simulink model "Final_EV_Model"  (R2020b)
settings: Solver=VariableStepAuto  StartTime=0.0  StopTime=2000  RelTol=1e-3
model workspace (MAT data in the model file):
  SoC_initial = Simulink.Parameter
  SoC_initial.DataType = 'auto'
  SoC_initial.Dimensions = [0 0]
values from neighbouring files (symbols this model uses):
  eff1 = [65 65 65 65 65 65 65 65 65 65 65 65 ... (600000 elements, 12000x50)]    [Frid27May_Data.mat]
  eff2 = [78 78 78 78 78 78 78 78 78 78 78 78 ... (600000 elements, 12000x50)]    [Frid27May_Data.mat]
  eff3 = [78 78 78 78 78 78 78 78 78 78 78 78 ... (600000 elements, 12000x50)]    [Frid27May_Data.mat]
  eff4 = [78 78 78 78 78 78 78 78 78 78 78 78 ... (600000 elements, 12000x50)]    [Frid27May_Data.mat]
  eff5 = [76 76 76 76 76 76 76 76 76 76 76 76 ... (600000 elements, 12000x50)]    [Frid27May_Data.mat]
  speed = [1 2 3 4 5 6 7 8 9 10 11 12 ... (12000 elements, 1x12000)]    [Frid27May_Data.mat]
  torque1 = [1 2 3 4 5 6 7 8 9 10 11 12 ... (50 elements, 1x50)]    [Frid27May_Data.mat]
  torque2 = [51 52 53 54 55 56 57 58 59 60 61 62 ... (50 elements, 1x50)]    [Frid27May_Data.mat]
  torque3 = [101 102 103 104 105 106 107 108 109 110 111 112 ... (50 elements, 1x50)]    [Frid27May_Data.mat]
  torque4 = [151 152 153 154 155 156 157 158 159 160 161 162 ... (50 elements, 1x50)]    [Frid27May_Data.mat]
  torque5 = [201 202 203 204 205 206 207 208 209 210 211 212 ... (50 elements, 1x50)]    [Frid27May_Data.mat]
undefined symbols (not defined in the file or in its folder): temp_inside, temp_outside
libraries: drivingcycle_lib x2, pid_lib x1
settings Model: Creator=joshuaafengbai  LastModifiedBy=joshuaafengbai

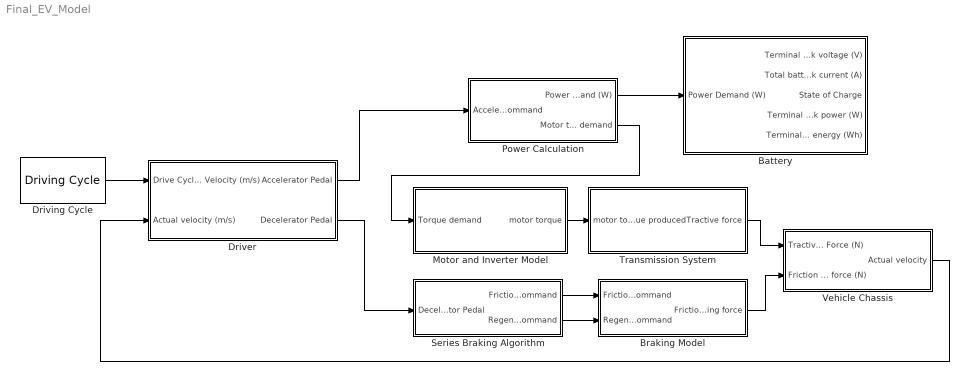
== system Final_EV_Model ==
  Battery : Subsystem
  Braking Model : Subsystem
  "Driver " : Subsystem
  Driving Cycle : drivingcycle_lib/Driving Cycle  CycleName=NEDC  CycleRepeatsForever=off
      settings: SourceProductName=Driving Cycle Blockset
  Motor and Inverter Model : Subsystem
  Power Calculation : Subsystem
  Series Braking Algorithm : Subsystem
  Transmission System : Subsystem
  Vehicle Chassis : Subsystem
  wires:
  Motor and Inverter Model/1(motor torque) -> Transmission System/1(motor torque produced)
  Transmission System/1(Tractive force) -> Vehicle Chassis/1(Tractive Force (N))
  "Driver "/1(Accelerator Pedal) -> Power Calculation/1(Acceleration command)
  Vehicle Chassis/1(Actual velocity) -> "Driver "/2(Actual velocity (m/s))
  Driving Cycle/2 -> "Driver "/1(Drive Cycle Velocity (m/s))
  "Driver "/2(Decelerator Pedal) -> Series Braking Algorithm/1(Decelerator Pedal)
  Series Braking Algorithm/1(" Friction brake command") -> Braking Model/1(Friction command)
  Series Braking Algorithm/2(Regen brake command) -> Braking Model/2(Regen command)
  Power Calculation/1(Power Demand (W)) -> Battery/1(Power Demand (W))
  Power Calculation/2(Motor torque demand) -> Motor and Inverter Model/1(Torque demand)
  Braking Model/1(Friction braking force) -> Vehicle Chassis/2(Friction braking force (N))

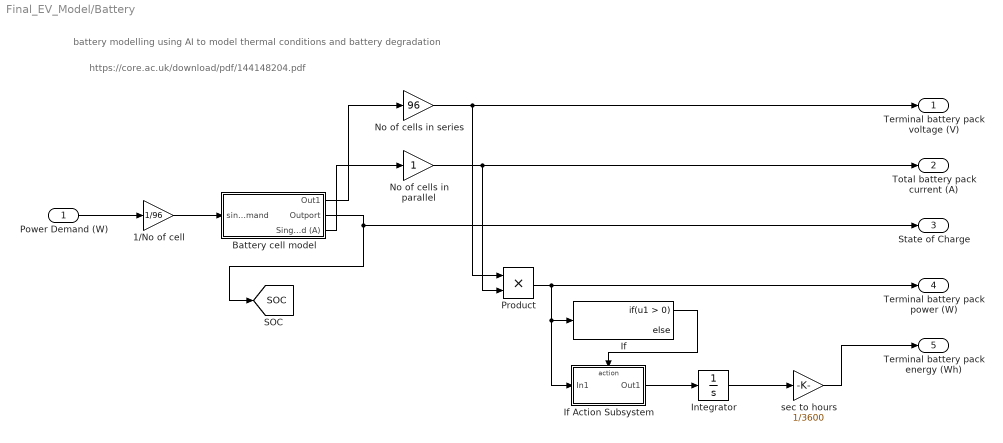
== system Final_EV_Model/Battery ==
  note: battery modelling using AI to model thermal conditions and battery degradation
  note: https://core.ac.uk/download/pdf/144148204.pdf
  Power Demand (W) : Inport
  1/No of cell : Gain  Gain=1/96
  Battery cell model : Subsystem
  If : If
  If Action Subsystem : Subsystem  TreatAsAtomicUnit=on
  Integrator : Integrator
  No of cells in parallel : Gain
  No of cells in series : Gain  Gain=96
  Product : Product
  sec to hours : Gain  Gain=1/3600
  Terminal battery pack voltage (V) : Outport
  Total battery pack current (A) : Outport  Port=2
  State of Charge : Outport  Port=3
  Terminal battery pack power (W) : Outport  Port=4
  Terminal battery pack energy (Wh) : Outport  Port=5
  tag scope: SOC=global
  wires:
  No of cells in series/1 -> Product/1, Terminal battery pack voltage (V)/1
  No of cells in parallel/1 -> Total battery pack current (A)/1, Product/2
  Product/1 -> If/1, If Action Subsystem/1(In1), Terminal battery pack power (W)/1
  sec to hours/1 -> Terminal battery pack energy (Wh)/1
  Integrator/1 -> sec to hours/1
  1/No of cell/1 -> Battery cell model/1(single cell power demand)
  Battery cell model/1(Out1) -> No of cells in series/1
  Battery cell model/2(Outport) -> State of Charge/1, [SOC]
  Power Demand (W)/1 -> 1/No of cell/1
  Battery cell model/3(Single cell current demand (A)) -> No of cells in parallel/1
  If/1 -> If Action Subsystem/Action
  If Action Subsystem/1(Out1) -> Integrator/1

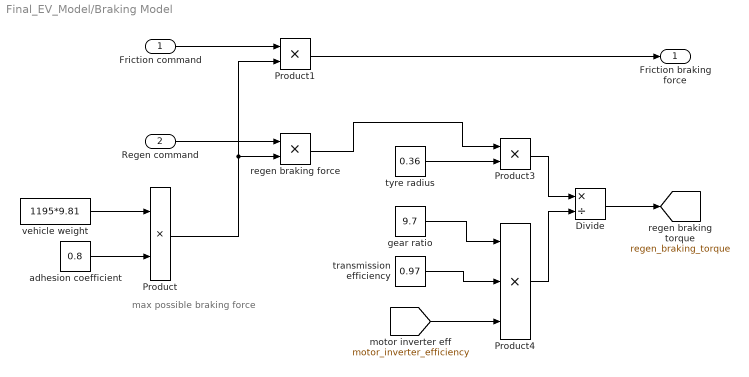
== system Final_EV_Model/Braking Model ==
  note: max possible
      | braking force
  Friction command : Inport
  Regen command : Inport  Port=2
  Divide : Product  Inputs=*/
  Product : Product
  Product1 : Product
  Product3 : Product
  Product4 : Product  Inputs=3
  adhesion coefficient : Constant  Value=0.8
  gear ratio : Constant  Value=9.7
  regen braking force : Product
  transmission efficiency : Constant  Value=0.97
  tyre radius : Constant  Value=0.36
  vehicle weight : Constant  Value=1195*9.81
  Friction braking force : Outport
  tag scope: regen_braking_torque=global
  wires:
  vehicle weight/1 -> Product/1
  adhesion coefficient/1 -> Product/2
  Product1/1 -> Friction braking force/1
  regen braking force/1 -> Product3/1
  Product/1 -> Product1/2, regen braking force/2
  Friction command/1 -> Product1/1
  Regen command/1 -> regen braking force/1
  tyre radius/1 -> Product3/2
  gear ratio/1 -> Product4/1
  transmission efficiency/1 -> Product4/2
  Product3/1 -> Divide/1
  Product4/1 -> Divide/2
  Divide/1 -> [regen_braking_torque]
  [motor_inverter_efficiency] -> Product4/3

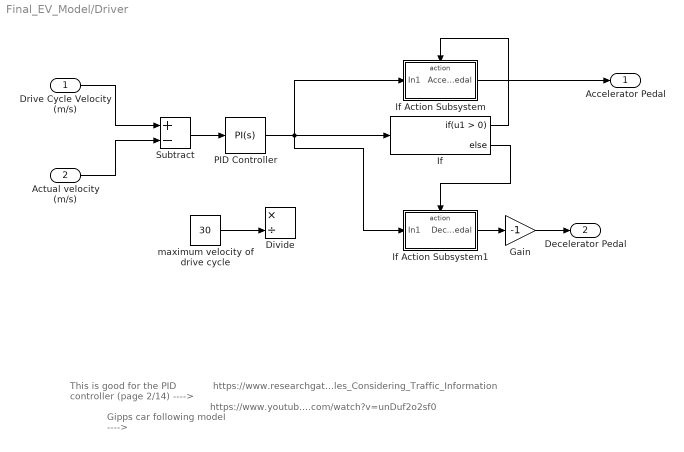
== system Final_EV_Model/Driver  ==
  note: Gipps car following model ---->
  note: https://www.youtube.com/watch?v=unDuf2o2sf0
  note: This is good for the PID controller (page 2/14) ---->
  note: https://www.researchgate.net/publication/335954963_Research_on_the_Energy-Saving_Strategy_of_Path_Planning_for_Electric_Vehicles_Considering_Traffic_Information
  Drive Cycle Velocity (m/s) : Inport
  Actual velocity (m/s) : Inport  Port=2
  Divide : Product  Inputs=*/
  Gain : Gain  Gain=-1
  If : If
  If Action Subsystem : Subsystem  TreatAsAtomicUnit=on
  If Action Subsystem1 : Subsystem  TreatAsAtomicUnit=on
  PID Controller : pid_lib/PID Controller  Controller=PI  Form=Parallel  TimeDomain=Continuous-time  UseExternalTs=off  SampleTime=-1  IntegratorMethod=Forward Euler  FilterMethod=Forward Euler  ControllerParametersSource=internal  P=10  I=1  D=0  UseFilter=on  N=1  TunerSelectOption=Transfer Function Based (PID Tuner App)  InitialConditionSource=internal  InitialConditionForIntegrator=0  InitialConditionForFilter=0  DifferentiatorICPrevScaledInput=0  ExternalReset=none  TrackingMode=off  Kt=1  LimitOutput=off  SatLimitsSource=internal  UpperSaturationLimit=inf  LowerSaturationLimit=-inf  LinearizeAsGain=on  AntiWindupMode=none  Kb=1  POutMin=[]  POutMax=[]  IOutMin=[]  IOutMax=[]  DOutMin=[]  DOutMax=[]  NOutMin=[]  NOutMax=[]  SumOutMin=[]  SumOutMax=[]  SaturationOutMin=[]  SaturationOutMax=[]  PParamMin=[]  PParamMax=[]  IParamMin=[]  IParamMax=[]  DParamMin=[]  DParamMax=[]  NParamMin=[]  NParamMax=[]  KbParamMin=[]  KbParamMax=[]  KtParamMin=[]  KtParamMax=[]  KbOutMin=[]  KbOutMax=[]  KtOutMin=[]  KtOutMax=[]  IntegratorOutMin=[]  IntegratorOutMax=[]  FilterOutMin=[]  FilterOutMax=[]  SumI1OutMin=[]  SumI1OutMax=[]  SumI2OutMin=[]  SumI2OutMax=[]  SumI3OutMin=[]  SumI3OutMax=[]  SumI4OutMin=[]  SumI4OutMax=[]  SumDOutMin=[]  SumDOutMax=[]  DifferentiatorOutMin=[]  DifferentiatorOutMax=[]  FilterDiffOutCoefMin=[]  FilterDiffOutCoefMax=[]  ReciprocalOutMin=[]  ReciprocalOutMax=[]  SumDenOutMin=[]  SumDenOutMax=[]  SumNumOutMin=[]  SumNumOutMax=[]  DivideOutMin=[]  DivideOutMax=[]  UdiffTsProdOutMin=[]  UdiffTsProdOutMax=[]  NTsProdOutMin=[]  NTsProdOutMax=[]  UintegralTsProdOutMin=[]  UintegralTsProdOutMax=[]  UngainTsProdOutMin=[]  UngainTsProdOutMax=[]  IntegratorContinuousStateAttributes=''  IntegratorStateMustResolveToSignalObject=off  IntegratorRTWStateStorageClass=Auto  FilterContinuousStateAttributes=''  FilterStateMustResolveToSignalObject=off  FilterRTWStateStorageClass=Auto  ParallelPVariant=InternalParameters  IdealPVariant=Disabled  IVariant=InternalParameters  DVariant=Disabled  IntegratorVariant=Continuous  SatVariant=Disabled  AWVariant=Passthrough  PCopyVariant=Disabled  TRVariant=Disabled  FdbkBlocksVariant=Forward  IdealPFdbkVariant=Disabled  SatFdbkVariant=Disabled  DerivativeFilterVariant=Disabled  NVariant=Disabled  NCopyVariant=Disabled_SignalSpec  FilterICVariant=Disabled  IntegratorICVariant=InternalICs  ExternalResetVariant=Disabled  TRSumVariant=Passthrough  SumFdbkVariant=Disabled  SumVariant=Sum_PI  TsampFilterVariant=InternalTs  TsampNgainVariant=Passthrough  TsampIntegralVariant=Passthrough  ExternalSaturationOutDataTypeStr=Inherit: Same as second input
  Subtract : Sum  Inputs=+-
  maximum velocity of drive cycle : Constant  Value=30
  Accelerator Pedal : Outport
  Decelerator Pedal : Outport  Port=2
  wires:
  Drive Cycle Velocity (m/s)/1 -> Subtract/1
  Actual velocity (m/s)/1 -> Subtract/2
  Subtract/1 -> PID Controller/1
  If/1 -> If Action Subsystem/Action
  If/2 -> If Action Subsystem1/Action
  maximum velocity of drive cycle/1 -> Divide/2
  If Action Subsystem/1(Accelerator Pedal) -> Accelerator Pedal/1
  PID Controller/1 -> If/1, If Action Subsystem/1(In1), If Action Subsystem1/1(In1)
  If Action Subsystem1/1(Decelerator Pedal) -> Gain/1
  Gain/1 -> Decelerator Pedal/1

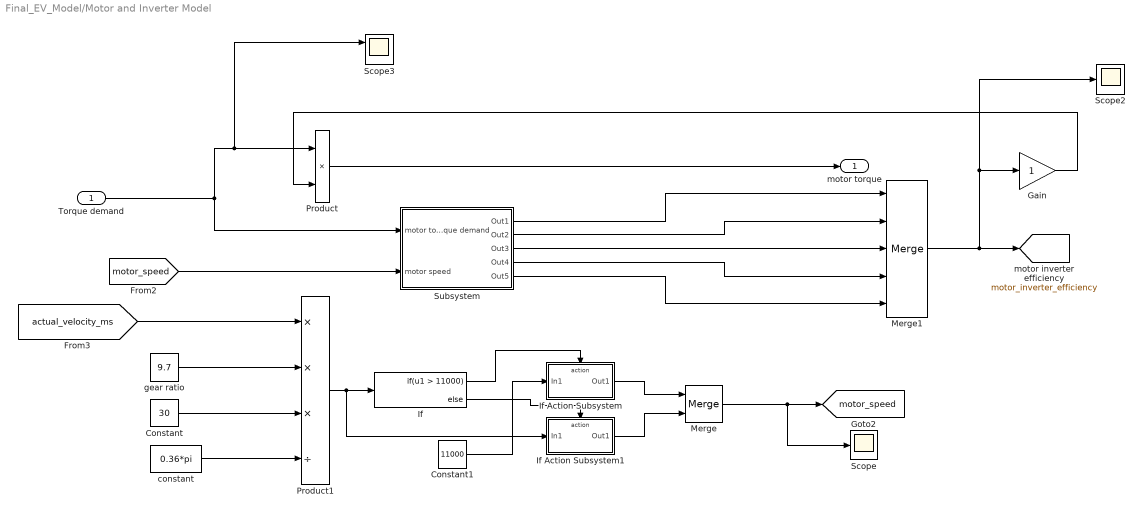
== system Final_EV_Model/Motor and Inverter Model ==
  Torque demand : Inport
  Constant : Constant  Value=30
  Constant1 : Constant  Value=11000
  Gain : Gain
  If : If  IfExpression=u1 > 11000
  If Action Subsystem : Subsystem  TreatAsAtomicUnit=on
  If Action Subsystem1 : Subsystem  TreatAsAtomicUnit=on
  Merge : Merge
  Merge1 : Merge  Inputs=5
  Product : Product
  Product1 : Product  Inputs=***/
  Scope : Scope
  Scope2 : Scope
  Scope3 : Scope  NumInputPorts=2
  Subsystem : Subsystem
  constant : Constant  Value=0.36*pi
  gear ratio : Constant  Value=9.7
  motor torque : Outport
  tag scope: motor_inverter_efficiency=global, motor_speed=global
  wires:
  Merge1/1 -> Scope2/1, Gain/1, [motor_inverter_efficiency]
  Product/1 -> motor torque/1
  [actual_velocity_ms] -> Product1/1
  gear ratio/1 -> Product1/2
  Torque demand/1 -> Scope3/1, Product/1, Subsystem/1(motor torque demand)
  [motor_speed] -> Subsystem/2(motor speed)
  Subsystem/1(Out1) -> Merge1/1
  Subsystem/2(Out2) -> Merge1/2
  Subsystem/3(Out3) -> Merge1/3
  Subsystem/4(Out4) -> Merge1/4
  Subsystem/5(Out5) -> Merge1/5
  Constant/1 -> Product1/3
  constant/1 -> Product1/4
  If/1 -> If Action Subsystem/Action
  Product1/1 -> If Action Subsystem1/1(In1), If/1
  Constant1/1 -> If Action Subsystem/1(In1)
  If/2 -> If Action Subsystem1/Action
  If Action Subsystem/1(Out1) -> Merge/1
  If Action Subsystem1/1(Out1) -> Merge/2
  Merge/1 -> Scope/1, [motor_speed]
  Gain/1 -> Product/2

== system Final_EV_Model/Power Calculation ==
  Acceleration command : Inport
  Add : Sum
  Add1 : Sum  Inputs=-+
  Gain : Gain  Gain=3/5
  Product : Product
  Scope : Scope
  auxillary system power demand : Subsystem
  driving power demand : Subsystem
  max available torque (Nm) : Constant  Value=250
  Power Demand (W) : Outport
  Motor torque demand : Outport  Port=2
  wires:
  Add/1 -> Power Demand (W)/1
  Acceleration command/1 -> Product/2
  Product/1 -> Motor torque demand/1, Add1/2
  auxillary system power demand/1(Power Demand (W)) -> Add/1
  Add1/1 -> driving power demand/1(Torque demand (Nm))
  driving power demand/1(power demand (W)) -> Add/2
  max available torque (Nm)/1 -> Product/1
  [regen_braking_torque] -> Gain/1
  Gain/1 -> Scope/1, Add1/1

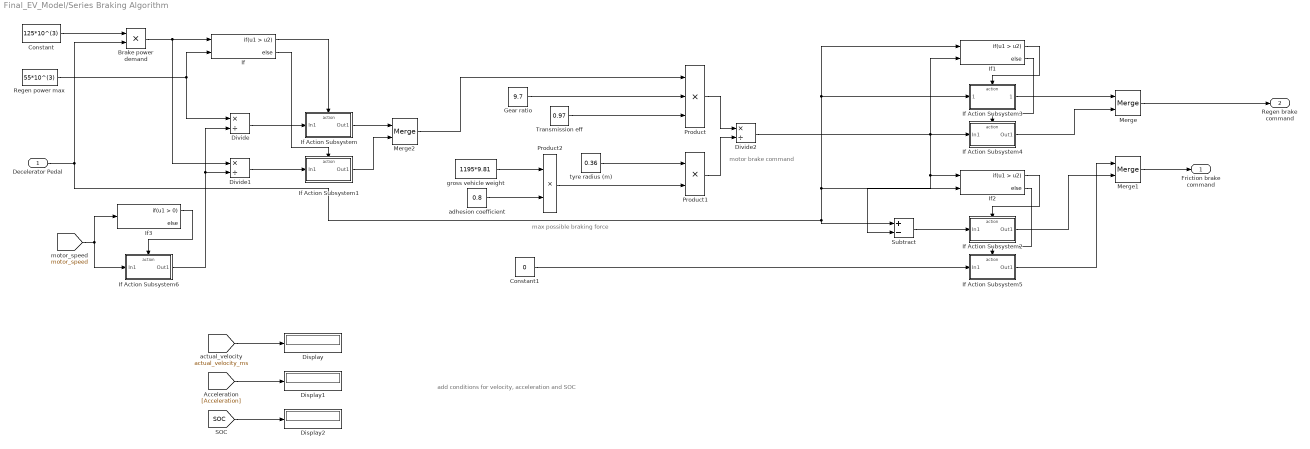
== system Final_EV_Model/Series Braking Algorithm ==
  note: add conditions for velocity, acceleration and SOC
  note: motor brake
      | command
  note: max possible
      | braking force
  Decelerator Pedal : Inport
  Brake power demand : Product
  Constant : Constant  Value=125*10^(3)
  Constant1 : Constant  Value=0
  Display : Display
  Display1 : Display
  Display2 : Display
  Divide : Product  Inputs=*/
  Divide1 : Product  Inputs=*/
  Divide2 : Product  Inputs=*/
  Gear ratio : Constant  Value=9.7
  If : If  NumInputs=2  IfExpression=u1 > u2
  If Action Subsystem : Subsystem  TreatAsAtomicUnit=on
  If Action Subsystem1 : Subsystem  TreatAsAtomicUnit=on
  If Action Subsystem2 : Subsystem  TreatAsAtomicUnit=on
  If Action Subsystem3 : Subsystem  TreatAsAtomicUnit=on
  If Action Subsystem4 : Subsystem  TreatAsAtomicUnit=on
  If Action Subsystem5 : Subsystem  TreatAsAtomicUnit=on
  If Action Subsystem6 : Subsystem  TreatAsAtomicUnit=on
  If1 : If  NumInputs=2  IfExpression=u1 > u2
  If2 : If  NumInputs=2  IfExpression=u1 > u2
  If3 : If
  Merge : Merge
  Merge1 : Merge
  Merge2 : Merge
  Product : Product  Inputs=3
  Product1 : Product
  Product2 : Product
  Regen power max : Constant  Value=55*10^(3)
  Subtract : Sum  Inputs=+-
  Transmission eff : Constant  Value=0.97
  adhesion coefficient : Constant  Value=0.8
  gross vehicle weight : Constant  Value=1195*9.81
  tyre radius (m) : Constant  Value=0.36
  " Friction brake command" : Outport
  Regen brake command : Outport  Port=2
  wires:
  Regen power max/1 -> Divide/1, If/2
  Brake power demand/1 -> If/1, Divide1/1
  If/1 -> If Action Subsystem/Action
  [motor_speed] -> If Action Subsystem6/1(In1), If3/1
  Divide/1 -> If Action Subsystem/1(In1)
  If/2 -> If Action Subsystem1/Action
  Divide1/1 -> If Action Subsystem1/1(In1)
  Gear ratio/1 -> Product/2
  Transmission eff/1 -> Product/3
  tyre radius (m)/1 -> Product1/1
  gross vehicle weight/1 -> Product2/1
  Product2/1 -> Product1/2
  adhesion coefficient/1 -> Product2/2
  Product/1 -> Divide2/1
  Product1/1 -> Divide2/2
  Decelerator Pedal/1 -> If1/1, If Action Subsystem3/1(Decelerator Pedal), If2/2, Subtract/1, Brake power demand/2
  Divide2/1 -> If1/2, If2/1, Subtract/2, If Action Subsystem4/1(In1)
  If1/1 -> If Action Subsystem3/Action
  If Action Subsystem3/1(Regen brake command) -> Merge/1
  If1/2 -> If Action Subsystem4/Action
  Constant1/1 -> If Action Subsystem5/1(In1)
  Subtract/1 -> If Action Subsystem2/1(In1)
  If Action Subsystem4/1(Out1) -> Merge/2
  If Action Subsystem5/1(Out1) -> Merge1/1
  If Action Subsystem2/1(Out1) -> Merge1/2
  Merge1/1 -> " Friction brake command"/1
  If Action Subsystem/1(Out1) -> Merge2/1
  If Action Subsystem1/1(Out1) -> Merge2/2
  Merge2/1 -> Product/1
  If2/1 -> If Action Subsystem2/Action
  If2/2 -> If Action Subsystem5/Action
  Constant/1 -> Brake power demand/1
  [SOC] -> Display2/1
  [Acceleration] -> Display1/1
  [actual_velocity_ms] -> Display/1
  If3/1 -> If Action Subsystem6/Action
  If Action Subsystem6/1(Out1) -> Divide1/2, Divide/2
  Merge/1 -> Regen brake command/1

== system Final_EV_Model/Transmission System ==
  motor torque produced : Inport
  Divide : Product  Inputs=*/
  Product : Product  Inputs=3
  Single speed gear ratio : Constant  Value=9.7
  dynamic tyre radius : Constant  Value=0.36
  transmission efficiency : Constant  Value=0.97
  Tractive force : Outport
  wires:
  motor torque produced/1 -> Product/1
  Single speed gear ratio/1 -> Product/2
  transmission efficiency/1 -> Product/3
  Product/1 -> Divide/1
  dynamic tyre radius/1 -> Divide/2
  Divide/1 -> Tractive force/1

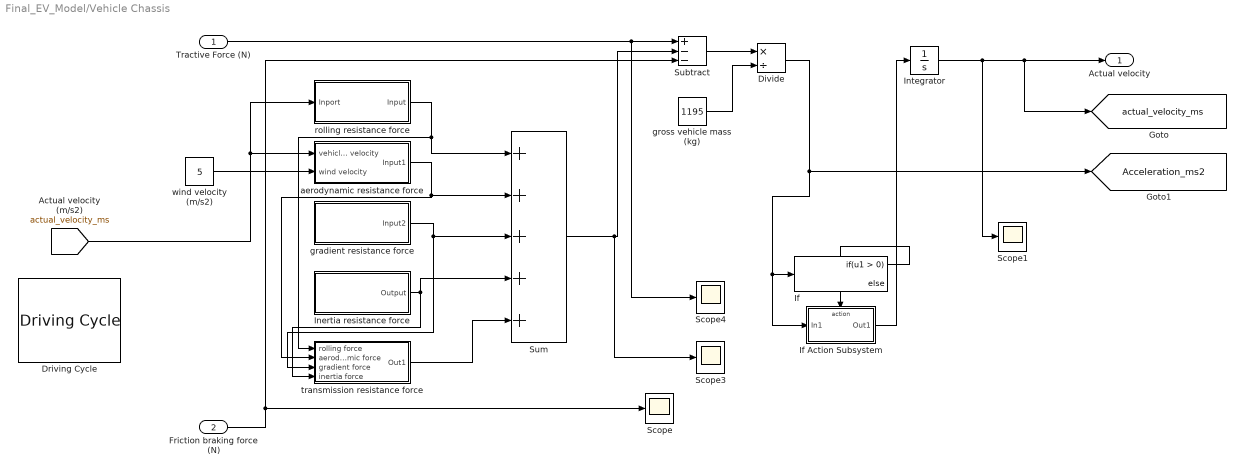
== system Final_EV_Model/Vehicle Chassis ==
  Tractive Force (N) : Inport
  Friction braking force (N) : Inport  Port=2
  Divide : Product  Inputs=*/
  Driving Cycle : drivingcycle_lib/Driving Cycle  CycleName=NEDC  CycleRepeatsForever=off
      settings: SourceProductName=Driving Cycle Blockset
  If : If
  If Action Subsystem : Subsystem  TreatAsAtomicUnit=on
  Inertia resistance force : Subsystem
  Integrator : Integrator
  Scope{,1,3..4} (4 alike) : Scope
  Subtract : Sum  Inputs=+--
  Sum : Sum  Inputs=5
  aerodynamic resistance force : Subsystem
  gradient resistance force : Subsystem
  gross vehicle mass (kg) : Constant  Value=1195
  rolling resistance force : Subsystem
  transmission resistance force : Subsystem
  wind velocity (m/s2) : Constant  Value=5
  Actual velocity : Outport
  tag scope: Acceleration_ms2=global, actual_velocity_ms=global
  wires:
  rolling resistance force/1(Input) -> Sum/1, transmission resistance force/1(rolling force)
  aerodynamic resistance force/1(Input1) -> transmission resistance force/2(aerodynamic force), Sum/2
  gradient resistance force/1(Input2) -> Sum/3, transmission resistance force/3(gradient force)
  Inertia resistance force/1(Output) -> Sum/4, transmission resistance force/4(inertia force)
  transmission resistance force/1(Out1) -> Sum/5
  Sum/1 -> Scope3/1, Subtract/2
  Subtract/1 -> Divide/1
  gross vehicle mass (kg)/1 -> Divide/2
  Divide/1 -> If Action Subsystem/1(In1), If/1, [Acceleration_ms2]
  Integrator/1 -> Scope1/1, [actual_velocity_ms], Actual velocity/1
  Friction braking force (N)/1 -> Scope/1, Subtract/3
  Tractive Force (N)/1 -> Scope4/1, Subtract/1
  wind velocity (m/s2)/1 -> aerodynamic resistance force/2(wind velocity)
  [actual_velocity_ms] -> rolling resistance force/1(Inport), aerodynamic resistance force/1(vehicle velocity)
  If/1 -> If Action Subsystem/Action
  If Action Subsystem/1(Out1) -> Integrator/1

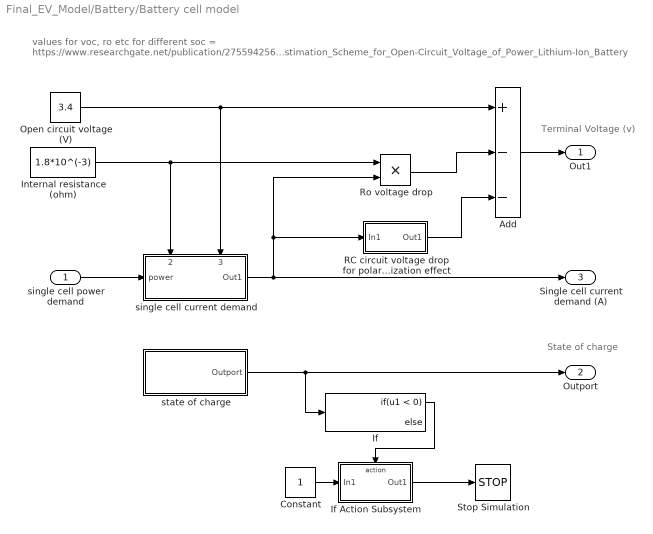
== system Final_EV_Model/Battery/Battery cell model ==
  note: values for voc, ro etc for different soc = https://www.researchgate.net/publication/275594256_An_Adaptive_Estimation_Scheme_for_Open-Circuit_Voltage_of_Power_Lithium-Ion_Battery
  note: State of charge
  note: Terminal Voltage (v)
  single cell power demand : Inport
  Add : Sum  Inputs=+--
  Constant : Constant
  If : If  IfExpression=u1 < 0
  If Action Subsystem : Subsystem  TreatAsAtomicUnit=on
  Internal resistance (ohm) : Constant  Value=1.8*10^(-3)
  Open circuit voltage (V) : Constant  Value=3.4
  RC circuit voltage drop for polarization effect : Subsystem
  Ro voltage drop : Product
  Stop Simulation : Stop
  single cell current demand : Subsystem
      settings: PortSchema="{\"entries\":[{\"content\":{\"sides\":[{\"content\":{\"connectorIds\":[\"In1\"]},\"type\":\"ConnectorPlacement.EquallySpacedRectSide\",\"uuid\":\"452fb404-3499-444b-bf84-c62c9102e51b\"},{\"content\":{\"connectorIds\":[\"Out1\"],\"side\":\"RIGHT\"},\"type\":\"ConnectorPlacement.EquallySpacedRectSide\",\"uuid\":\"cda393a8-5c39-4647-8a74-a8f2574f759a\"},{\"content\":{\"connectorIds\":[\"In2\",\"In3\"],\"side\":\"TOP\"},\"type\":\"ConnectorPlacement.EquallySpacedRectSide\",\"uuid\":\"c10ce816-4b9a-41d0-a449-ee0f20672a9d\"},{\"content\":{\"connectorIds\":[],\"side\":\"HIDDEN\"},\"type\":\"ConnectorPlacement.EquallySpacedRectSide\",\"uuid\":\"fadcce9a-a202-4481-8868-e19c169caf1d\"}]},\"type\":\"ConnectorPlacement.EquallySpacedConnector\",\"uuid\":\"f11ce6f4-0652-4898-ba48-baa514fa4dd7\"}],\"packageUris\":[\"http://schema.mathworks.com/mf0/Connector/R2020b\"],\"version\":\"1.0\"}"
  state of charge : Subsystem
  Out1 : Outport
  Outport : Outport  Port=2
  Single cell current demand (A) : Outport  Port=3
  wires:
  Ro voltage drop/1 -> Add/2
  Internal resistance (ohm)/1 -> single cell current demand/2(single cell current), Ro voltage drop/1
  Open circuit voltage (V)/1 -> single cell current demand/3(open circuit voltage), Add/1
  Add/1 -> Out1/1
  single cell current demand/1(Out1) -> Single cell current demand (A)/1, Ro voltage drop/2, RC circuit voltage drop for polarization effect/1(In1)
  single cell power demand/1 -> single cell current demand/1(power)
  RC circuit voltage drop for polarization effect/1(Out1) -> Add/3
  If/1 -> If Action Subsystem/Action
  Constant/1 -> If Action Subsystem/1(In1)
  state of charge/1(Outport) -> If/1, Outport/1
  If Action Subsystem/1(Out1) -> Stop Simulation/1

== system Final_EV_Model/Battery/If Action Subsystem ==
  In1 : Inport
  Action Port : ActionPort  ActionPortLabel=if(u1 > 0)
  Out1 : Outport
  wires:
  In1/1 -> Out1/1

== system Final_EV_Model/Driver /If Action Subsystem ==
  In1 : Inport
  Action Port : ActionPort  ActionPortLabel=if(u1 > 0)
  Accelerator Pedal : Outport
  wires:
  In1/1 -> Accelerator Pedal/1

== system Final_EV_Model/Driver /If Action Subsystem1 ==
  In1 : Inport
  Action Port : ActionPort  ActionPortLabel=else
  Decelerator Pedal : Outport
  wires:
  In1/1 -> Decelerator Pedal/1

== system Final_EV_Model/Motor and Inverter Model/If Action Subsystem ==
  In1 : Inport
  Action Port : ActionPort  ActionPortLabel=if(u1 > 11000)
  Out1 : Outport
  wires:
  In1/1 -> Out1/1

== system Final_EV_Model/Motor and Inverter Model/If Action Subsystem1 ==
  In1 : Inport
  Action Port : ActionPort  ActionPortLabel=else
  Out1 : Outport
  wires:
  In1/1 -> Out1/1

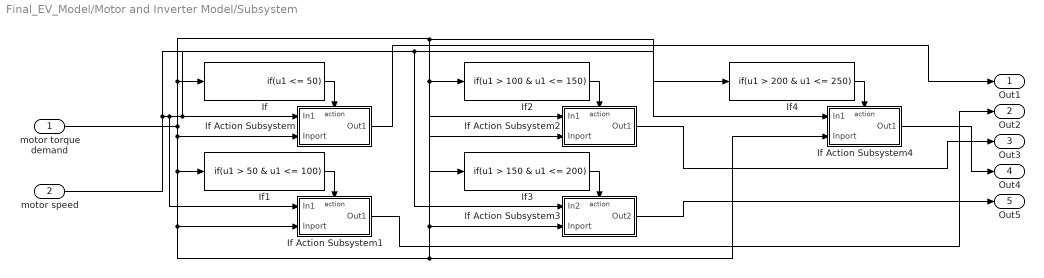
== system Final_EV_Model/Motor and Inverter Model/Subsystem ==
  motor torque demand : Inport
  motor speed : Inport  Port=2
  If : If  IfExpression=u1 <= 50  ShowElse=off
  If Action Subsystem : Subsystem  TreatAsAtomicUnit=on
  If Action Subsystem1 : Subsystem  TreatAsAtomicUnit=on
  If Action Subsystem2 : Subsystem  TreatAsAtomicUnit=on
  If Action Subsystem3 : Subsystem  TreatAsAtomicUnit=on
  If Action Subsystem4 : Subsystem  TreatAsAtomicUnit=on
  If1 : If  IfExpression=u1 > 50 & u1 <= 100  ShowElse=off
  If2 : If  IfExpression=u1 > 100 & u1 <= 150  ShowElse=off
  If3 : If  IfExpression=u1 > 150 & u1 <= 200  ShowElse=off
  If4 : If  IfExpression=u1 > 200 & u1 <= 250  ShowElse=off
  Out1 : Outport
  Out2 : Outport  Port=2
  Out3 : Outport  Port=3
  Out4 : Outport  Port=4
  Out5 : Outport  Port=5
  wires:
  If Action Subsystem4/1(Out1) -> Out4/1
  If Action Subsystem2/1(Out1) -> Out3/1
  If1/1 -> If Action Subsystem1/Action
  If Action Subsystem/1(Out1) -> Out1/1
  motor speed/1 -> If Action Subsystem3/1(In2), If Action Subsystem2/1(In1), If Action Subsystem/1(In1), If Action Subsystem4/1(In1), If Action Subsystem1/1(In1)
  If4/1 -> If Action Subsystem4/Action
  If Action Subsystem1/1(Out1) -> Out2/1
  If3/1 -> If Action Subsystem3/Action
  If2/1 -> If Action Subsystem2/Action
  If Action Subsystem3/1(Out2) -> Out5/1
  If/1 -> If Action Subsystem/Action
  motor torque demand/1 -> If1/1, If Action Subsystem1/2(Inport), If Action Subsystem4/2(Inport), If Action Subsystem3/2(Inport), If Action Subsystem2/2(Inport), If Action Subsystem/2(Inport), If4/1, If2/1, If3/1, If/1

== system Final_EV_Model/Power Calculation/auxillary system power demand ==
  note: on or off depending on driving cycle
  note: on or off depending on driving cycle
  note: on or off depending on driving cycle
  12V battery eff : Constant  Value=0.9
  Add : Sum  Inputs=++++++
  DC/DC converter eff : Constant  Value=0.9
  Divide : Product  Inputs=*/
  Driving Control : Constant  Value=150
  Energy Management System : Constant  Value=150
  HVAC Power Demand : Subsystem  Commented=on
  Head and Tail Lamps : Constant  Value=150
  Power Steering : Constant  Value=400
  Product : Product
  Power Demand (W) : Outport
  wires:
  Driving Control/1 -> Add/4
  Energy Management System/1 -> Add/5
  Head and Tail Lamps/1 -> Add/6
  Add/1 -> Divide/1
  Product/1 -> Divide/2
  Divide/1 -> Power Demand (W)/1
  DC/DC converter eff/1 -> Product/1
  12V battery eff/1 -> Product/2

== system Final_EV_Model/Power Calculation/driving power demand ==
  Torque demand (Nm) : Inport
  If : If  IfExpression=u1 > 125000
  If Action Subsystem : Subsystem  TreatAsAtomicUnit=on
  If Action Subsystem1 : Subsystem  TreatAsAtomicUnit=on
  If Action Subsystem2 : Subsystem  TreatAsAtomicUnit=on
  If1 : If
  Merge : Merge
  Product : Product
  Scope : Scope
  max power demand : Constant  Value=125000
  power demand (W) : Outport
  wires:
  Torque demand (Nm)/1 -> Product/2
  [motor_speed] -> Product/1
  If/1 -> If Action Subsystem/Action
  If Action Subsystem/1(Out1) -> Merge/2
  Merge/1 -> power demand (W)/1
  max power demand/1 -> If Action Subsystem/1(In1)
  If/2 -> If Action Subsystem1/Action
  If Action Subsystem1/1(Out1) -> Merge/1
  Product/1 -> Scope/1, If Action Subsystem2/1(In1), If1/1
  If1/1 -> If Action Subsystem2/Action
  If Action Subsystem2/1(Out1) -> If Action Subsystem1/1(In1), If/1

== system Final_EV_Model/Series Braking Algorithm/If Action Subsystem ==
  In1 : Inport
  Action Port : ActionPort  ActionPortLabel=if(u1 > u2)
  Out1 : Outport
  wires:
  In1/1 -> Out1/1

== system Final_EV_Model/Series Braking Algorithm/If Action Subsystem1 ==
  In1 : Inport
  Action Port : ActionPort  ActionPortLabel=else
  Out1 : Outport
  wires:
  In1/1 -> Out1/1

== system Final_EV_Model/Series Braking Algorithm/If Action Subsystem2 ==
  In1 : Inport
  Action Port : ActionPort  ActionPortLabel=if(u1 > u2)
  Out1 : Outport
  wires:
  In1/1 -> Out1/1

== system Final_EV_Model/Series Braking Algorithm/If Action Subsystem3 ==
  Decelerator Pedal : Inport
  Action Port : ActionPort  ActionPortLabel=if(u1 > u2)
  Regen brake command : Outport
  wires:
  Decelerator Pedal/1 -> Regen brake command/1

== system Final_EV_Model/Series Braking Algorithm/If Action Subsystem4 ==
  In1 : Inport
  Action Port : ActionPort  ActionPortLabel=else
  Out1 : Outport
  wires:
  In1/1 -> Out1/1

== system Final_EV_Model/Series Braking Algorithm/If Action Subsystem5 ==
  In1 : Inport
  Action Port : ActionPort  ActionPortLabel=else
  Out1 : Outport
  wires:
  In1/1 -> Out1/1

== system Final_EV_Model/Series Braking Algorithm/If Action Subsystem6 ==
  In1 : Inport
  Action Port : ActionPort  ActionPortLabel=if(u1 > 0)
  Out1 : Outport
  wires:
  In1/1 -> Out1/1

== system Final_EV_Model/Vehicle Chassis/If Action Subsystem ==
  In1 : Inport
  Action Port : ActionPort  ActionPortLabel=if(u1 > 0)
  Out1 : Outport
  wires:
  In1/1 -> Out1/1

== system Final_EV_Model/Vehicle Chassis/Inertia resistance force ==
  Abs : Abs
  Coefficient of rotary inertia : Constant  Value=1.15
  Constant : Constant
  Product : Product  Inputs=3
  Scope : Scope
  gross vehicle mass : Constant  Value=1195
  Output : Outport
  wires:
  Coefficient of rotary inertia/1 -> Product/1
  gross vehicle mass/1 -> Product/2
  Product/1 -> Abs/1, Scope/1
  Constant/1 -> Product/3
  Abs/1 -> Output/1

== system Final_EV_Model/Vehicle Chassis/aerodynamic resistance force ==
  vehicle velocity : Inport
  wind velocity : Inport  Port=2
  Constant : Constant  Value=0.5
  Display : Display
  Frontal area : Constant  Value=2.38
  Product : Product  Inputs=5
  Scope : Scope
  Square : Math  Operator=square  SaturateOnIntegerOverflow=on
  Subtract : Sum  Inputs=+-
  coefficient of drag : Constant  Value=0.22
  rho : Constant  Value=1.225
  Input1 : Outport
  wires:
  Constant/1 -> Product/1
  Frontal area/1 -> Product/2
  rho/1 -> Product/3
  coefficient of drag/1 -> Product/4
  Square/1 -> Product/5
  Product/1 -> Scope/1, Display/1, Input1/1
  Subtract/1 -> Square/1
  vehicle velocity/1 -> Subtract/1
  wind velocity/1 -> Subtract/2

== system Final_EV_Model/Vehicle Chassis/gradient resistance force ==
  Display : Display
  Product : Product
  Sin : Trigonometry
  gross vehicle weight : Constant  Value=1195*9.81
  slope angle theta (in rad) : Constant  Value=0
  Input2 : Outport
  wires:
  Product/1 -> Display/1, Input2/1
  slope angle theta (in rad)/1 -> Sin/1
  Sin/1 -> Product/2
  gross vehicle weight/1 -> Product/1

== system Final_EV_Model/Vehicle Chassis/rolling resistance force ==
  note: coefficient of rolling force calculation
  Inport : Inport
  Add : Sum
  Constant : Constant  Value=100
  Constant1 : Constant
  Constant2 : Constant  Value=0.01
  Display : Display
  Divide : Product  Inputs=*/
  Product : Product
  Product1 : Product
  Scope : Scope
  gross vehicle weight : Constant  Value=1195*9.81
  Input : Outport
  wires:
  gross vehicle weight/1 -> Product/1
  Product/1 -> Scope/1, Display/1, Input/1
  Inport/1 -> Divide/1
  Constant/1 -> Divide/2
  Divide/1 -> Add/1
  Constant1/1 -> Add/2
  Constant2/1 -> Product1/1
  Add/1 -> Product1/2
  Product1/1 -> Product/2

== system Final_EV_Model/Vehicle Chassis/transmission resistance force ==
  rolling force : Inport
  aerodynamic force : Inport  Port=2
  gradient force : Inport  Port=3
  inertia force : Inport  Port=4
  1-transmission eff : Constant  Value=0.03
  Divide : Product  Inputs=**/
  Scope : Scope
  Sum : Sum  Inputs=|++++
  transmission eff : Constant  Value=0.97
  Out1 : Outport
  wires:
  rolling force/1 -> Sum/1
  aerodynamic force/1 -> Sum/2
  gradient force/1 -> Sum/3
  inertia force/1 -> Sum/4
  transmission eff/1 -> Divide/3
  Divide/1 -> Scope/1, Out1/1
  Sum/1 -> Divide/2
  1-transmission eff/1 -> Divide/1

== system Final_EV_Model/Battery/Battery cell model/If Action Subsystem ==
  In1 : Inport
  Action Port : ActionPort  ActionPortLabel=if(u1 < 0)
  Out1 : Outport
  wires:
  In1/1 -> Out1/1

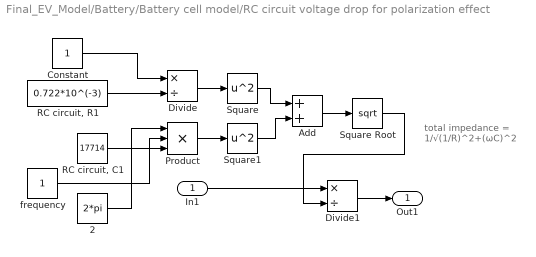
== system Final_EV_Model/Battery/Battery cell model/RC circuit voltage drop for polarization effect ==
  note: total impedance =
      |
      | 1/√(1/R)^2+(ωC)^2
  In1 : Inport
  2 : Constant  Value=2*pi
  Add : Sum
  Constant : Constant
  Divide : Product  Inputs=*/
  Divide1 : Product  Inputs=*/
  Product : Product  Inputs=3
  "RC circuit, C1" : Constant  Value=17714
  "RC circuit, R1" : Constant  Value=0.722*10^(-3)
  Square : Math  Operator=square  SaturateOnIntegerOverflow=on
  Square Root : Sqrt  SaturateOnIntegerOverflow=on
  Square1 : Math  Operator=square  SaturateOnIntegerOverflow=on
  frequency : Constant
  Out1 : Outport
  wires:
  "RC circuit, R1"/1 -> Divide/2
  Constant/1 -> Divide/1
  Divide/1 -> Square/1
  "RC circuit, C1"/1 -> Product/3
  2/1 -> Product/1
  frequency/1 -> Product/2
  Product/1 -> Square1/1
  Square/1 -> Add/1
  Square1/1 -> Add/2
  Add/1 -> Square Root/1
  Divide1/1 -> Out1/1
  In1/1 -> Divide1/1
  Square Root/1 -> Divide1/2

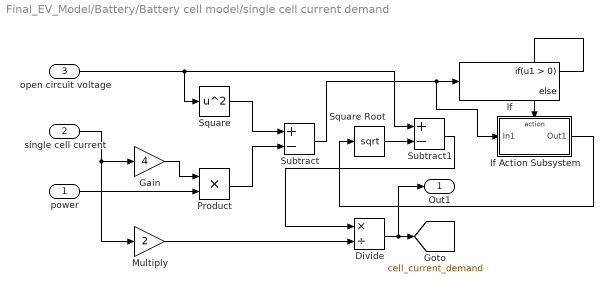
== system Final_EV_Model/Battery/Battery cell model/single cell current demand ==
  power : Inport
  single cell current : Inport  Port=2
  open circuit voltage : Inport  Port=3
  Divide : Product  Inputs=*/
  Gain : Gain  Gain=4
  If : If
  If Action Subsystem : Subsystem  TreatAsAtomicUnit=on
  Multiply : Gain  Gain=2
  Product : Product
  Square : Math  Operator=square  SaturateOnIntegerOverflow=on
  Square Root : Sqrt  SaturateOnIntegerOverflow=on
  Subtract : Sum  Inputs=+-
  Subtract1 : Sum  Inputs=+-
  Out1 : Outport
  tag scope: cell_current_demand=global
  wires:
  Multiply/1 -> Divide/2
  Divide/1 -> Out1/1, [cell_current_demand]
  Product/1 -> Subtract/2
  Square/1 -> Subtract/1
  Gain/1 -> Product/1
  single cell current/1 -> Gain/1, Multiply/1
  Subtract1/1 -> Divide/1
  open circuit voltage/1 -> Subtract1/1, Square/1
  Square Root/1 -> Subtract1/2
  Subtract/1 -> If Action Subsystem/1(In1), If/1
  power/1 -> Product/2
  If/1 -> If Action Subsystem/Action
  If Action Subsystem/1(Out1) -> Square Root/1

== system Final_EV_Model/Battery/Battery cell model/state of charge ==
  Divide : Product  Inputs=*/
  If : If
  If Action Subsystem : Subsystem  TreatAsAtomicUnit=on
  Integrator : Integrator
  Scope : Scope
  Single cell capacity (Ah) : Constant  Value=60
  Subtract : Sum  Inputs=+-
  soc_initial : Constant  Value=100
  Outport : Outport
  wires:
  soc_initial/1 -> Subtract/1
  Divide/1 -> Integrator/1
  Integrator/1 -> Subtract/2
  Subtract/1 -> Outport/1
  [cell_current_demand] -> If/1, If Action Subsystem/1(In1)
  If/1 -> If Action Subsystem/Action
  If Action Subsystem/1(Out1) -> Scope/1, Divide/1
  Single cell capacity (Ah)/1 -> Divide/2

== system Final_EV_Model/Motor and Inverter Model/Subsystem/If Action Subsystem ==
  In1 : Inport
  Inport : Inport  Port=2
  Action Port : ActionPort  ActionPortLabel=if(u1 <= 50)
  1-D Lookup Table1 : Lookup_n-D  BreakpointsForDimension1=speed  BreakpointsForDimension2=torque1  BreakpointsForDimension3=[1:5]  Table=eff1  InternalRulePriority=Speed  RndMeth=Simplest  InputSameDT=on
      settings: InputPortMap=u0,u1
  Out1 : Outport
  wires:
  In1/1 -> 1-D Lookup Table1/1
  Inport/1 -> 1-D Lookup Table1/2
  1-D Lookup Table1/1 -> Out1/1

== system Final_EV_Model/Motor and Inverter Model/Subsystem/If Action Subsystem1 ==
  In1 : Inport
  Inport : Inport  Port=2
  Action Port : ActionPort  ActionPortLabel=if(u1 > 50 & u1 <= 100)
  1-D Lookup Table1 : Lookup_n-D  BreakpointsForDimension1=speed  BreakpointsForDimension2=torque2  BreakpointsForDimension3=[1:5]  Table=eff2  InternalRulePriority=Speed  RndMeth=Simplest  InputSameDT=on
      settings: InputPortMap=u0,u1
  Out1 : Outport
  wires:
  In1/1 -> 1-D Lookup Table1/1
  Inport/1 -> 1-D Lookup Table1/2
  1-D Lookup Table1/1 -> Out1/1

== system Final_EV_Model/Motor and Inverter Model/Subsystem/If Action Subsystem2 ==
  In1 : Inport
  Inport : Inport  Port=2
  Action Port : ActionPort  ActionPortLabel=if(u1 > 100 & u1 <= 150)
  1-D Lookup Table1 : Lookup_n-D  BreakpointsForDimension1=speed  BreakpointsForDimension2=torque3  BreakpointsForDimension3=[1:5]  Table=eff3  InternalRulePriority=Speed  RndMeth=Simplest  InputSameDT=on
      settings: InputPortMap=u0,u1
  Out1 : Outport
  wires:
  In1/1 -> 1-D Lookup Table1/1
  Inport/1 -> 1-D Lookup Table1/2
  1-D Lookup Table1/1 -> Out1/1

== system Final_EV_Model/Motor and Inverter Model/Subsystem/If Action Subsystem3 ==
  In2 : Inport
  Inport : Inport  Port=2
  Action Port : ActionPort  ActionPortLabel=if(u1 > 150 & u1 <= 200)
  1-D Lookup Table1 : Lookup_n-D  BreakpointsForDimension1=speed  BreakpointsForDimension2=torque4  BreakpointsForDimension3=[1:5]  Table=eff4  InternalRulePriority=Speed  RndMeth=Simplest  InputSameDT=on
      settings: InputPortMap=u0,u1
  Out2 : Outport
  wires:
  In2/1 -> 1-D Lookup Table1/1
  Inport/1 -> 1-D Lookup Table1/2
  1-D Lookup Table1/1 -> Out2/1

== system Final_EV_Model/Motor and Inverter Model/Subsystem/If Action Subsystem4 ==
  In1 : Inport
  Inport : Inport  Port=2
  Action Port : ActionPort  ActionPortLabel=if(u1 > 200 & u1 <= 250)
  1-D Lookup Table1 : Lookup_n-D  BreakpointsForDimension1=speed  BreakpointsForDimension2=torque5  BreakpointsForDimension3=[1:5]  Table=eff5  InternalRulePriority=Speed  RndMeth=Simplest  InputSameDT=on
      settings: InputPortMap=u0,u1
  Out1 : Outport
  wires:
  In1/1 -> 1-D Lookup Table1/1
  Inport/1 -> 1-D Lookup Table1/2
  1-D Lookup Table1/1 -> Out1/1

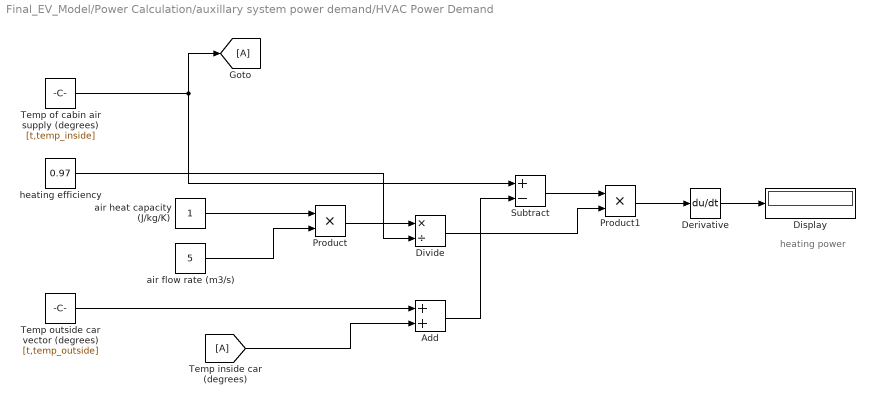
== system Final_EV_Model/Power Calculation/auxillary system power demand/HVAC Power Demand ==
  note: heating power
  Add : Sum
  Derivative : Derivative
  Display : Display
  Divide : Product  Inputs=*/
  Product : Product
  Product1 : Product
  Subtract : Sum  Inputs=+-
  Temp of cabin air supply (degrees) : Constant  Value=[t,temp_inside]
  Temp outside car vector (degrees) : Constant  Value=[t,temp_outside]
  air flow rate (m3/s) : Constant  Value=5
  air heat capacity (J/kg/K) : Constant
  heating efficiency : Constant  Value=0.97
  wires:
  Divide/1 -> Product1/2
  Temp outside car vector (degrees)/1 -> Add/1
  Temp of cabin air supply (degrees)/1 -> Subtract/1, [A]
  [A] -> Add/2
  Product1/1 -> Derivative/1
  heating efficiency/1 -> Divide/2
  air flow rate (m3/s)/1 -> Product/2
  Subtract/1 -> Product1/1
  air heat capacity (J/kg/K)/1 -> Product/1
  Product/1 -> Divide/1
  Derivative/1 -> Display/1
  Add/1 -> Subtract/2

== system Final_EV_Model/Power Calculation/driving power demand/If Action Subsystem ==
  In1 : Inport
  Action Port : ActionPort  ActionPortLabel=if(u1 > 125000)
  Out1 : Outport
  wires:
  In1/1 -> Out1/1

== system Final_EV_Model/Power Calculation/driving power demand/If Action Subsystem1 ==
  In1 : Inport
  Action Port : ActionPort  ActionPortLabel=else
  Out1 : Outport
  wires:
  In1/1 -> Out1/1

== system Final_EV_Model/Power Calculation/driving power demand/If Action Subsystem2 ==
  In1 : Inport
  Action Port : ActionPort  ActionPortLabel=if(u1 > 0)
  Out1 : Outport
  wires:
  In1/1 -> Out1/1

== system Final_EV_Model/Battery/Battery cell model/single cell current demand/If Action Subsystem ==
  In1 : Inport
  Action Port : ActionPort  ActionPortLabel=if(u1 > 0)
  Out1 : Outport
  wires:
  In1/1 -> Out1/1

== system Final_EV_Model/Battery/Battery cell model/state of charge/If Action Subsystem ==
  In1 : Inport
  Action Port : ActionPort  ActionPortLabel=if(u1 > 0)
  Out1 : Outport
  wires:
  In1/1 -> Out1/1
